simulink model "EngPrt_OvrSpd"  (R2016b)
settings: configuration reference "CodeGenConfigSet" (kept outside this file)
values from neighbouring files (symbols this model uses):
  EngPrt_nOvrSpd_C = Calibration.Parameter    [init_EngPrt_OvrSpd.m]    (also in init_EngPrt_OvrSpd_SIL.m = Simulink.Parameter)
  EngPrt_tiOvrSpdDeb_C = Calibration.Parameter    [init_EngPrt_OvrSpd.m]    (also in init_EngPrt_OvrSpd_SIL.m = Simulink.Parameter)
undefined symbols (not defined in the file or in its folder): EngPrt_OvrSpd_DT
libraries: CXLib x3
settings Model: Creator=Administrator  LastModifiedBy=Administrator
settings ConfigSetRef: SourceLocation=Base Workspace

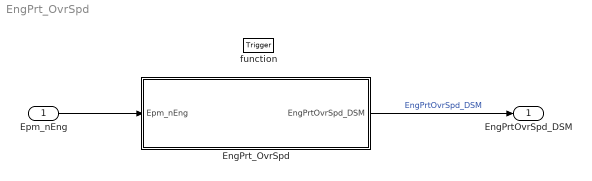
== system EngPrt_OvrSpd ==
  Epm_nEng : Inport  Tag=rpm  Description=Engine speed  OutMin=0  OutMax=6000  OutDataTypeStr=EngSpeed_rpm
  function : TriggerPort  TriggerType=function-call  VariantControl=Variant
  EngPrt_OvrSpd : Subsystem
  EngPrtOvrSpd_DSM : Outport  Description=Diagnostic Fault Check for overspeed detection  OutMin=0  OutMax=1  OutDataTypeStr=boolean
  wires:
  Epm_nEng/1 -> EngPrt_OvrSpd/1(Epm_nEng)
  EngPrt_OvrSpd/1(EngPrtOvrSpd_DSM) -> EngPrtOvrSpd_DSM/1  "EngPrtOvrSpd_DSM"

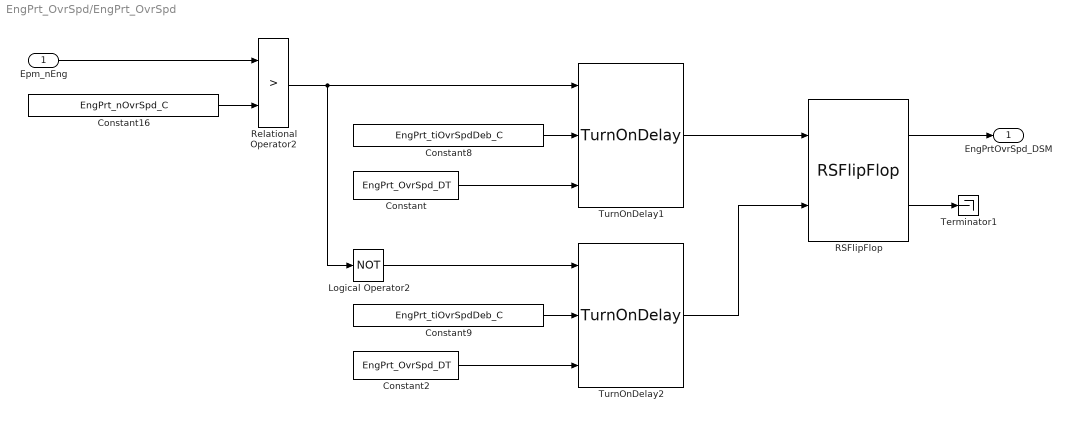
== system EngPrt_OvrSpd/EngPrt_OvrSpd ==
  Epm_nEng : Inport  Tag=rpm  Description=Engine Speed  OutMin=0  OutMax=6000  OutDataTypeStr=EngSpeed_rpm
  Constant : Constant  Value=EngPrt_OvrSpd_DT  OutDataTypeStr=Inherit: Inherit via back propagation
  Constant16 : Constant  Value=EngPrt_nOvrSpd_C
  Constant2 : Constant  Value=EngPrt_OvrSpd_DT  OutDataTypeStr=Inherit: Inherit via back propagation
  Constant8 : Constant  Value=EngPrt_tiOvrSpdDeb_C
  Constant9 : Constant  Value=EngPrt_tiOvrSpdDeb_C
  Logical Operator2 : Logic  Operator=NOT  AllPortsSameDT=off  OutDataTypeStr=boolean
  RSFlipFlop : CXLib/RSFlipFlop
  Relational Operator2 : RelationalOperator  Operator=>  OutDataTypeStr=boolean  RndMeth=Nearest  InputSameDT=on
  Terminator1 : Terminator
  TurnOnDelay1 : CXLib/TurnOnDelay
  TurnOnDelay2 : CXLib/TurnOnDelay
  EngPrtOvrSpd_DSM : Outport
  wires:
  Logical Operator2/1 -> TurnOnDelay2/1
  Constant9/1 -> TurnOnDelay2/2
  Relational Operator2/1 -> Logical Operator2/1, TurnOnDelay1/1
  Constant16/1 -> Relational Operator2/2
  Epm_nEng/1 -> Relational Operator2/1
  Constant/1 -> TurnOnDelay1/3
  Constant8/1 -> TurnOnDelay1/2
  Constant2/1 -> TurnOnDelay2/3
  TurnOnDelay1/1 -> RSFlipFlop/1
  TurnOnDelay2/1 -> RSFlipFlop/2
  RSFlipFlop/2 -> Terminator1/1
  RSFlipFlop/1 -> EngPrtOvrSpd_DSM/1
